simulink model "EV3_pos_control"  (Simulink 7.6)
settings: Solver=FixedStepDiscrete  StartTime=0.0  StopTime=Inf  RelTol=1e-3
InitFcn:
  | nxt_rst
undefined symbols (not defined in the file): S, Te
libraries: rpi_blkst x1
settings Model: Creator=jacques  LastModifiedBy=jacques  SimulationMode=external
settings OptimizationCC: OptimizeModelRefInitCode=on  LifeSpan=1
settings HardwareCC: ProdLargestAtomicInteger=Long  ProdLargestAtomicFloat=Double  ProdEndianess=LittleEndian  ProdHWDeviceType=ARM Compatible->ARM 11
settings RTWCC: SystemTargetFile=ert_rpi.tlc  TemplateMakefile=ert_rpi.tmf  PostCodeGenCommand=postGenFunc(buildInfo)  Description=RTW Embedded Coder RPI target  ProcessScript=ert_rpi_make_rtw_hook
settings CodeAppCC: IgnoreCustomStorageClasses=off
settings STFCustomTargetCC: ModelReferenceCompliant=off  CombineOutputUpdateFcns=on  ERTCustomFileBanners=on  SupportNonInlinedSFcns=off  SystemTargetFile=ert_rpi.tlc
settings ERTTargetCC: MultiwordLength=2048  ModelReferenceCompliant=off  ParMdlRefBuildCompliant=off  CompOptLevelCompliant=off  ERTFirstTimeCompliant=off  SupportContinuousTime=on  ModelStepFunctionPrototypeControlCompliant=off  CPPClassGenCompliant=off  ExtMode=on  ExtModeMexArgs='192.168.2.1'  InlinedParameterPlacement=NonHierarchical  ERTCustomFileTemplate=ert_rpi_file_process.tlc  ConvertIfToSwitch=off

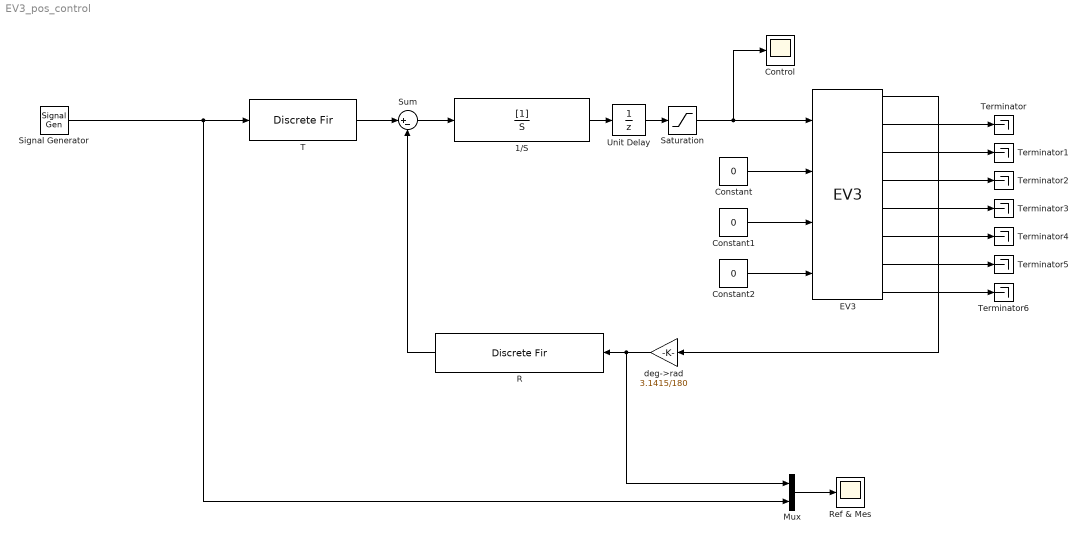
== system EV3_pos_control ==
  1/S : DiscreteFilter  Denominator=S  SampleTime=Te
  Constant : Constant  Value=0  SampleTime=0.01
  Constant1 : Constant  Value=0  SampleTime=0.01
  Constant2 : Constant  Value=0  SampleTime=0.01
  Control : Scope
      settings: YMin=-100  YMax=100
  EV3 : rpi_blkst/EV3  SystemSampleTime=-1  rpi_mask_Ts=Te
  Mux : Mux  Inputs=2
  R : DiscreteFir  NumCoeffs=R  SampleTime=Te
  Ref & Mes : Scope
      settings: YMin=-1  YMax=1
  Saturation : Saturate  UpperLimit=100  LowerLimit=-100  SampleTime=Te
  Signal Generator : SignalGenerator  Amplitude=0  Frequency=0.5
  Sum : Sum  Inputs=|+-
  T : DiscreteFir  NumCoeffs=T  SampleTime=Te
  Terminator{,1..6} (7 alike) : Terminator
  Unit Delay : UnitDelay  SampleTime=Te
  deg->rad : Gain  Gain=3.1415/180  SampleTime=Te
  wires:
  T/1 -> Sum/1
  R/1 -> Sum/2
  deg->rad/1 -> R/1, Mux/1
  Sum/1 -> 1/S/1
  1/S/1 -> Unit Delay/1
  Saturation/1 -> Control/1, EV3/1
  EV3/1 -> deg->rad/1
  Signal Generator/1 -> T/1, Mux/2
  EV3/2 -> Terminator/1
  EV3/3 -> Terminator1/1
  EV3/4 -> Terminator2/1
  EV3/5 -> Terminator3/1
  EV3/6 -> Terminator4/1
  EV3/7 -> Terminator5/1
  EV3/8 -> Terminator6/1
  Constant/1 -> EV3/2
  Constant1/1 -> EV3/3
  Constant2/1 -> EV3/4
  Mux/1 -> Ref & Mes/1
  Unit Delay/1 -> Saturation/1
